simulink model "DTCFinal"  (R2017b)
settings: Solver=FixedStepDiscrete  StartTime=0.0  StopTime=60  FixedStep=Ts  MaxStep=Ts  RelTol=1e-3  EnableMultiTasking=on
InitFcn:
  | Vdc=560;Ts=2e-5;wb=2*pi*50;Rr=2.486;
  | Rs=4.125;Lls=0.01557;Llr=0.01557;Lm=0.2848;
  | Xls=4.8915;
  | Xlr=4.8915;
  | Xm=89.4726;
  | Xml=2.3807;
  | P=4;
  | J=0.139;
  | 
  | Kp=8;
  | Ki=35;
  | Tlim=15;
  | 
  | fc=3800;
  | F=0.001;
undefined symbols (not defined in the file): DiscIntNeverNeededParam
libraries: simulink x5, eeGeneralControl x2, powerlib x1
settings Model: Creator=Lenovo  LastModifiedBy=M.H
settings OptimizationCC: LifeSpan=inf
settings DebuggingCC: SFUnexpectedBacktrackingDiag=warning  SFNoUnconditionalDefaultTransitionDiag=warning  SFExecutionAtInitializationDiag=none
settings CodeAppCC: StateflowObjectComments=on
settings GRTTargetCC: TargetLangStandard=C89/C90 (ANSI)  GeneratePreprocessorConditionals=Disable all
settings ConfigComp: CovMetricSettings=dw  CovHtmlReporting=on  CovSaveCumulativeToWorkspaceVar=on  CovSaveSingleToWorkspaceVar=on  CovExternalEMLEnable=off

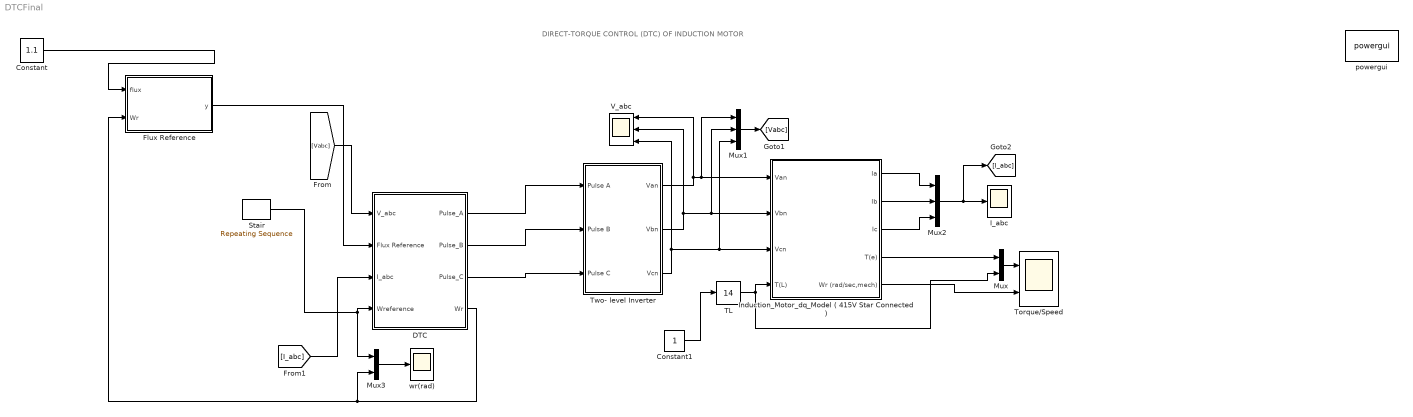
== system DTCFinal ==
  note: DIRECT-TORQUE CONTROL (DTC)
      | OF INDUCTION MOTOR
  Constant : Constant  Value=1.1
  Constant1 : Constant
  DTC : Subsystem
  Flux Reference : MATLAB Function  TreatAsAtomicUnit=on
  I_abc : Scope
  Induction_Motor_dq_Model ( 415V Star Connected ) : Subsystem
  Mux : Mux  Inputs=2
  Mux1 : Mux  Inputs=3
  Mux2 : Mux  Inputs=3
  Mux3 : Mux  Inputs=2
  "Stair " : simulink/Sources/Repeating Sequence  rep_seq_t=[0 0.1 0.11 4 4.1 8 8.1 12 12.1 16 18 19 20 22 22.5 23 25 26 29 30 35 40 50 55 60]  rep_seq_y=[0 0 10 10 20 20 30 30 40 40 60 80 100 110 120 130 140 150 160 170 200 300 400 400 400]
  TL : simulink/Math Operations/Slider Gain  gain=14  low=-14  high=14
  Torque/Speed : Scope  NumInputPorts=2
  "Two- level Inverter " : Subsystem
  V_abc : Scope  NumInputPorts=3
  powergui : powerlib/powergui  Priority=1  SimulationMode=Discrete  SampleTime=Ts  frequency=60  Iterations=50  frequencyindice=60  Pbase=100e6  ErrMax=1e-4  UnitsV=kV  UnitsW=MW  buscounter=0  FunctionMessages=off  echomessages=off  EnableUseOfTLC=off  CurrentSourceSwitches=off  DisableSnubberDevices=off  DisableRonSwitches=off  DisableVfSwitches=off  DisplayEquations=off  SolverType=Tustin/Backward Euler (TBE)  Interpol=off  ExternalGateDelay=off  methode=off  Ts=10  x0status=blocks  SPID=off  SwTol=0  HookPort=off  RestoreLinks=warning  ResistiveCurrentMeasurement=off  Frange=[0:2:500]  Ylog=off  Xlog=on  ShowGrid=off  save=off  variable=ZData  structure=ScopeData1  ZoomFFT=on  StartTime=0.0  cycles=4  DisplayStyle=2  fundamental=50  FreqAxis=off  MaxFrequency=1000  frequencyindicesteady=1  RmsSteady=1  display=off
  wr(rad) : Scope
  wires:
  Induction_Motor_dq_Model ( 415V Star Connected )/1(Ia) -> Mux2/1
  Induction_Motor_dq_Model ( 415V Star Connected )/2(Ib) -> Mux2/2
  Induction_Motor_dq_Model ( 415V Star Connected )/3(Ic) -> Mux2/3
  Induction_Motor_dq_Model ( 415V Star Connected )/5(Wr (rad/sec,mech)) -> Torque/Speed/2
  "Two- level Inverter "/1(Van) -> V_abc/1, Mux1/1, Induction_Motor_dq_Model ( 415V Star Connected )/1(Van)
  "Two- level Inverter "/3(Vcn) -> V_abc/3, Mux1/3, Induction_Motor_dq_Model ( 415V Star Connected )/3(Vcn)
  "Two- level Inverter "/2(Vbn) -> V_abc/2, Mux1/2, Induction_Motor_dq_Model ( 415V Star Connected )/2(Vbn)
  TL/1 -> Mux/2, Induction_Motor_dq_Model ( 415V Star Connected )/4(T(L))
  Constant1/1 -> TL/1
  Induction_Motor_dq_Model ( 415V Star Connected )/4(T(e)) -> Mux/1
  Mux/1 -> Torque/Speed/1
  Mux2/1 -> [I_abc], I_abc/1
  DTC/1(Pulse_A) -> "Two- level Inverter "/1(Pulse A)
  DTC/3(Pulse_C) -> "Two- level Inverter "/3(Pulse C)
  DTC/2(Pulse_B) -> "Two- level Inverter "/2(Pulse B)
  Mux1/1 -> [Vabc]
  Mux3/1 -> wr(rad)/1
  [Vabc] -> DTC/1(V_abc)
  [I_abc] -> DTC/3(I_abc)
  Flux Reference/1(y) -> DTC/2(Flux Reference)
  DTC/4(Wr) -> Flux Reference/2(Wr), Mux3/2
  Constant/1 -> Flux Reference/1(flux)
  "Stair "/1 -> Mux3/1, DTC/4(Wreference)

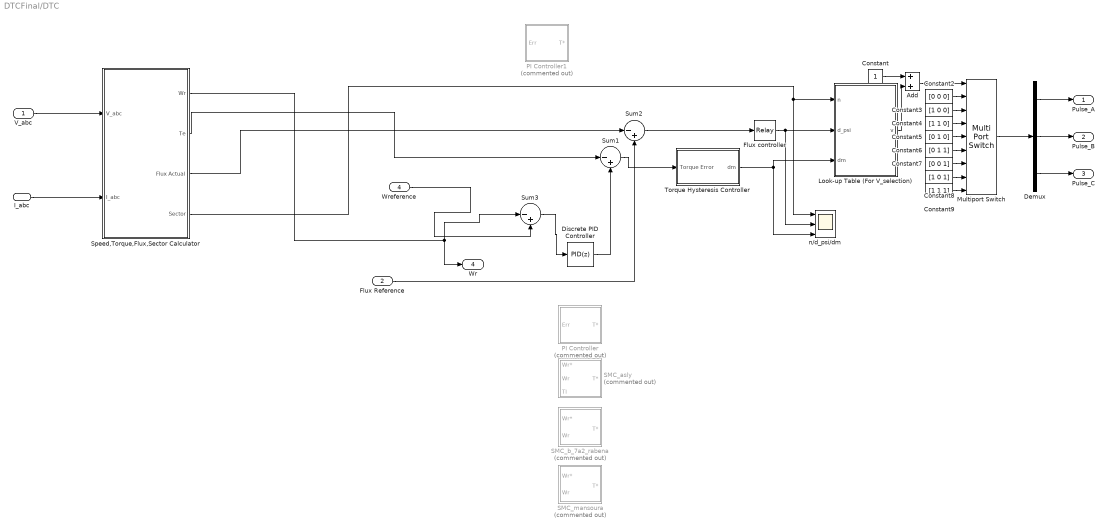
== system DTCFinal/DTC ==
  V_abc : Inport
  Flux Reference : Inport  Port=2
  I_abc : Inport  Port=3
  Wreference : Inport  Port=4
  Add : Sum
  Constant : Constant
  Constant2 : Constant  Value=[0 0 0]
  Constant3 : Constant  Value=[1 0 0]
  Constant4 : Constant  Value=[1 1 0]
  Constant5 : Constant  Value=[0 1 0]
  Constant6 : Constant  Value=[0 1 1]
  Constant7 : Constant  Value=[0 0 1]
  Constant8 : Constant  Value=[1 0 1]
  Constant9 : Constant  Value=[1 1 1]
  Demux : Demux  Outputs=3
  Discrete PID Controller : simulink/Continuous/PID Controller  Controller=PID  TimeDomain=Discrete-time  SampleTime=-1  IntegratorMethod=Forward Euler  FilterMethod=Forward Euler  Form=Parallel  UseFilter=on  ControllerParametersSource=internal  P=10  I=2  D=0  N=100  InitialConditionSource=internal  InitialConditionForIntegrator=0  InitialConditionForFilter=0  ExternalReset=none  LimitOutput=off  UpperSaturationLimit=inf  LowerSaturationLimit=-inf  LinearizeAsGain=off  AntiWindupMode=none  Kb=1  TrackingMode=off  Kt=1  PParamMin=[]  PParamMax=[]  IParamMin=[]  IParamMax=[]  DParamMin=[]  DParamMax=[]  NParamMin=[]  NParamMax=[]  KbParamMin=[]  KbParamMax=[]  KtParamMin=[]  KtParamMax=[]  POutMin=[]  POutMax=[]  IOutMin=[]  IOutMax=[]  DOutMin=[]  DOutMax=[]  NOutMin=[]  NOutMax=[]  KbOutMin=[]  KbOutMax=[]  KtOutMin=[]  KtOutMax=[]  IntegratorOutMin=[]  IntegratorOutMax=[]  FilterOutMin=[]  FilterOutMax=[]  SumOutMin=[]  SumOutMax=[]  SumI1OutMin=[]  SumI1OutMax=[]  SumI2OutMin=[]  SumI2OutMax=[]  SumI3OutMin=[]  SumI3OutMax=[]  SumDOutMin=[]  SumDOutMax=[]  SaturationOutMin=[]  SaturationOutMax=[]  IntegratorContinuousStateAttributes=''  IntegratorStateMustResolveToSignalObject=off  IntegratorRTWStateStorageClass=Auto  FilterContinuousStateAttributes=''  FilterStateMustResolveToSignalObject=off  FilterRTWStateStorageClass=Auto  DifferentiatorICPrevScaledInput=0  DifferentiatorOutMin=[]  DifferentiatorOutMax=[]  InitialConditionSetting=State (most efficient)  FilterDiffOutCoefMin=[]  FilterDiffOutCoefMax=[]  SumDenOutMin=[]  SumDenOutMax=[]  SumNumOutMin=[]  SumNumOutMax=[]  ReciprocalOutMin=[]  ReciprocalOutMax=[]  DivideOutMin=[]  DivideOutMax=[]  TunerSelectOption=Transfer Function Based (PID Tuner App)
  Flux controller : Relay  OnSwitchValue=0.02  OffSwitchValue=-0.02
  Look-up Table (For V_selection) : MATLAB Function  TreatAsAtomicUnit=on
  Multiport Switch : MultiPortSwitch  Inputs=8
  PI Controller : Subsystem  Commented=on
  PI Controller1 : Subsystem  Commented=on
  "SMC_asly " : Subsystem  Commented=on
  "SMC_b_7a2_rabena " : Subsystem  Commented=on
  "SMC_mansoura " : Subsystem  Commented=on
  Speed,Torque,Flux,Sector Calculator : Subsystem
  Sum1 : Sum  Inputs=|-+
  Sum2 : Sum  Inputs=|-+
  Sum3 : Sum  Inputs=|-+
  Torque Hysteresis Controller : Subsystem
  n/d_psi/dm : Scope  NumInputPorts=3
  Pulse_A : Outport
  Pulse_B : Outport  Port=2
  Pulse_C : Outport  Port=3
  Wr : Outport  Port=4
  wires:
  Flux controller/1 -> Look-up Table (For V_selection)/2(d_psi), n/d_psi/dm/2
  Sum2/1 -> Flux controller/1
  Speed,Torque,Flux,Sector Calculator/4(Sector) -> n/d_psi/dm/1, Look-up Table (For V_selection)/1(n)
  Torque Hysteresis Controller/1(dm) -> Look-up Table (For V_selection)/3(dm), n/d_psi/dm/3
  Flux Reference/1 -> Sum2/2
  Add/1 -> Multiport Switch/1
  Sum1/1 -> Torque Hysteresis Controller/1(Torque Error)
  Constant9/1 -> Multiport Switch/9
  Constant6/1 -> Multiport Switch/6
  Constant2/1 -> Multiport Switch/2
  Constant3/1 -> Multiport Switch/3
  Constant5/1 -> Multiport Switch/5
  Demux/3 -> Pulse_C/1
  Constant8/1 -> Multiport Switch/8
  Look-up Table (For V_selection)/1(v) -> Add/2
  Constant/1 -> Add/1
  Demux/1 -> Pulse_A/1
  Demux/2 -> Pulse_B/1
  Constant7/1 -> Multiport Switch/7
  Constant4/1 -> Multiport Switch/4
  Multiport Switch/1 -> Demux/1
  V_abc/1 -> Speed,Torque,Flux,Sector Calculator/1(V_abc)
  I_abc/1 -> Speed,Torque,Flux,Sector Calculator/2(I_abc)
  Speed,Torque,Flux,Sector Calculator/2(Te) -> Sum1/1
  Speed,Torque,Flux,Sector Calculator/3(Flux Actual) -> Sum2/1
  Speed,Torque,Flux,Sector Calculator/1(Wr) -> Sum3/1, Wr/1
  Wreference/1 -> Sum3/2
  Sum3/1 -> Discrete PID Controller/1
  Discrete PID Controller/1 -> Sum1/2

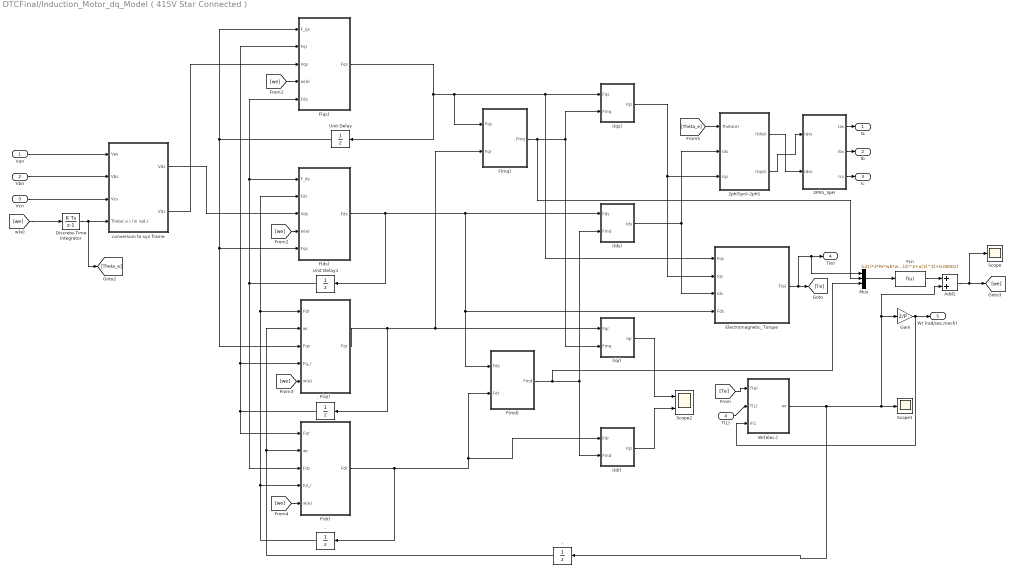
== system DTCFinal/Induction_Motor_dq_Model ( 415V Star Connected ) ==
  Van : Inport
  Vbn : Inport  Port=2
  Vcn : Inport  Port=3
  T(L) : Inport  Port=4
  . : UnitDelay  SampleTime=Ts
  ". " : UnitDelay  SampleTime=Ts
  ".  " : UnitDelay  SampleTime=Ts
  2PhS_3pH : Subsystem
  2ph(Syn)-2phS : Subsystem
  Add1 : Sum
  Discrete-Time Integrator : DiscreteIntegrator  InitialConditionSetting=State (most efficient)  SampleTime=Ts  ICPrevOutput=DiscIntNeverNeededParam  ICPrevScaledInput=DiscIntNeverNeededParam
  Electromagnetic_Torque : Subsystem
  F(dr) : Subsystem
  F(ds) : Subsystem
  F(md) : Subsystem
  F(mq) : Subsystem
  F(qr) : Subsystem
  F(qs) : Subsystem
  Fcn : Fcn  Expr=(u(1)*2*Rr*wb*wb)/(3*P*(u(2)^2+u(3)^2)+0.00001)
  Gain : Gain  Gain=2/P
  I(dr) : Subsystem
  I(ds) : Subsystem
  I(qr) : Subsystem
  I(qs) : Subsystem
  Mux : Mux  Inputs=3
  Scope : Scope
  Scope1 : Scope
  Scope2 : Scope  NumInputPorts=2
  Unit Delay : UnitDelay  SampleTime=Ts
  Unit Delay1 : UnitDelay  SampleTime=Ts
  Wr(elec.) : Subsystem
  "conversion to syn frame " : Subsystem
  Ia : Outport
  Ib : Outport  Port=2
  Ic : Outport  Port=3
  T(e) : Outport  Port=4
  Wr (rad/sec,mech) : Outport  Port=5
  wires:
  F(mq)/1(Fmq) -> Mux/2, I(qs)/2(Fmq), I(qr)/2(Fmq)
  I(ds)/1(Ids) -> Electromagnetic_Torque/3(Ids), 2ph(Syn)-2phS/2(Ids)
  I(qs)/1(Iqs) -> Electromagnetic_Torque/2(Iqs), 2ph(Syn)-2phS/3(Iqs)
  Wr(elec.)/1(wr) -> Scope1/1, Gain/1, Add1/2, ".  "/1
  Van/1 -> "conversion to syn frame "/1(Vas)
  I(dr)/1(Iqs) -> Scope2/2
  "conversion to syn frame "/1(Vds) -> F(ds)/3(Vds)
  Vcn/1 -> "conversion to syn frame "/3(Vcs)
  Vbn/1 -> "conversion to syn frame "/2(Vbs)
  "conversion to syn frame "/2(Vqs) -> F(qs)/3(Vqs)
  F(dr)/1(Fdr) -> ". "/1, F(md)/2(Fdr), I(dr)/1("Fdr ")
  F(ds)/1(Fds) -> Unit Delay1/1, I(ds)/1("Fds "), Electromagnetic_Torque/4(Fds), F(md)/1(Fds)
  F(qr)/1(Fqr) -> ./1, I(qr)/1("Fqr "), F(mq)/2(Fqr)
  I(qr)/1(Iqr) -> Scope2/1
  2ph(Syn)-2phS/1(I(dss)) -> 2PhS_3pH/2(Idss)
  2ph(Syn)-2phS/2(I(qss)) -> 2PhS_3pH/1(Iqss)
  F(qs)/1(Fqs) -> Unit Delay/1, Electromagnetic_Torque/1(Fqs), I(qs)/1("Fqs "), F(mq)/1(Fqs)
  [we] -> Discrete-Time Integrator/1
  [Theta_e] -> 2ph(Syn)-2phS/1(Theta(e))
  [we] -> F(dr)/5(w(e))
  Electromagnetic_Torque/1(T(e)) -> Mux/1, T(e)/1, [Te]
  2PhS_3pH/3(Ics) -> Ic/1
  T(L)/1 -> Wr(elec.)/2(T(L))
  2PhS_3pH/1(Ias) -> Ia/1
  2PhS_3pH/2(Ibs) -> Ib/1
  [we] -> F(qs)/4("w(e) ")
  [Te] -> Wr(elec.)/1(T(e))
  [we] -> F(qr)/5(w(e))
  [we] -> F(ds)/4("w(e) ")
  Discrete-Time Integrator/1 -> "conversion to syn frame "/4("Theta( e ) (in rad.) "), [Theta_e]
  Unit Delay/1 -> F(qs)/1(F_qs), F(ds)/5(Fqs), F(qr)/3(Fqs)
  Unit Delay1/1 -> F(ds)/1(F_ds), F(qs)/5(Fds), F(dr)/3(Fds)
  ./1 -> F(dr)/1(Fqr), F(qr)/4(Fq_r), F(qs)/2(Fqr)
  ". "/1 -> F(ds)/2(Fdr), F(qr)/1(Fdr), F(dr)/4(Fd_r)
  ".  "/1 -> F(qr)/2(wr), F(dr)/2(wr)
  F(md)/1(Fmd) -> Mux/3, I(ds)/2(Fmd), I(dr)/2(Fmd)
  Fcn/1 -> Add1/1
  Add1/1 -> Scope/1, [we]
  Mux/1 -> Fcn/1
  Gain/1 -> Wr(elec.)/3(In1), Wr (rad/sec,mech)/1

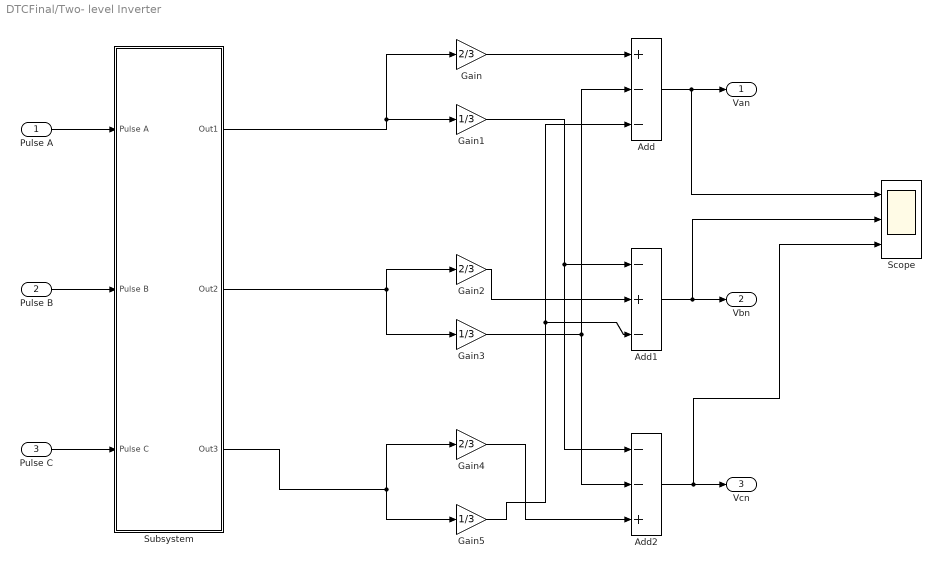
== system DTCFinal/Two- level Inverter  ==
  Pulse A : Inport
  Pulse B : Inport  Port=2
  Pulse C : Inport  Port=3
  Add : Sum  Inputs=+--
  Add1 : Sum  Inputs=-+-
  Add2 : Sum  Inputs=--+
  Gain : Gain  Gain=2/3
  Gain1 : Gain  Gain=1/3
  Gain2 : Gain  Gain=2/3
  Gain3 : Gain  Gain=1/3
  Gain4 : Gain  Gain=2/3
  Gain5 : Gain  Gain=1/3
  Scope : Scope  NumInputPorts=3
  Subsystem : Subsystem
  Van : Outport
  Vbn : Outport  Port=2
  Vcn : Outport  Port=3
  wires:
  Pulse C/1 -> Subsystem/3(Pulse C)
  Pulse B/1 -> Subsystem/2(Pulse B)
  Pulse A/1 -> Subsystem/1(Pulse A)
  Subsystem/2(Out2) -> Gain3/1, Gain2/1
  Subsystem/3(Out3) -> Gain4/1, Gain5/1
  Subsystem/1(Out1) -> Gain1/1, Gain/1
  Gain4/1 -> Add2/3
  Add/1 -> Scope/1, Van/1
  Add2/1 -> Vcn/1, Scope/3
  Gain3/1 -> Add/2, Add2/2
  Add1/1 -> Vbn/1, Scope/2
  Gain5/1 -> Add1/3, Add/3
  Gain/1 -> Add/1
  Gain2/1 -> Add1/2
  Gain1/1 -> Add1/1, Add2/1

== system DTCFinal/DTC/PI Controller ==
  Err : Inport
  "Integrator " : DiscreteIntegrator  InitialConditionSetting=State (most efficient)  SampleTime=Ts  LimitOutput=on  UpperSaturationLimit=Tlim  LowerSaturationLimit=-Tlim  ICPrevOutput=DiscIntNeverNeededParam  ICPrevScaledInput=DiscIntNeverNeededParam
  Ki : Gain  Gain=Ki
  Kp : Gain  Gain=Kp
  Saturation : Saturate  UpperLimit=Tlim  LowerLimit=-Tlim
  Sum1 : Sum  Inputs=|++
  T* : Outport
  wires:
  Err/1 -> Ki/1, Kp/1
  Ki/1 -> "Integrator "/1
  Kp/1 -> Sum1/1
  "Integrator "/1 -> Sum1/2
  Sum1/1 -> Saturation/1
  Saturation/1 -> T*/1

== system DTCFinal/DTC/PI Controller1 ==
  Err : Inport
  "Integrator " : DiscreteIntegrator  InitialConditionSetting=State (most efficient)  SampleTime=Ts  LimitOutput=on  UpperSaturationLimit=Tlim  LowerSaturationLimit=-Tlim  ICPrevOutput=DiscIntNeverNeededParam  ICPrevScaledInput=DiscIntNeverNeededParam
  Ki : Gain  Gain=Ki
  Kp : Gain  Gain=Kp
  Saturation : Saturate  UpperLimit=Tlim  LowerLimit=-Tlim
  Sum1 : Sum  Inputs=|++
  T* : Outport
  wires:
  Err/1 -> Ki/1, Kp/1
  Ki/1 -> "Integrator "/1
  Kp/1 -> Sum1/1
  "Integrator "/1 -> Sum1/2
  Sum1/1 -> Saturation/1
  Saturation/1 -> T*/1

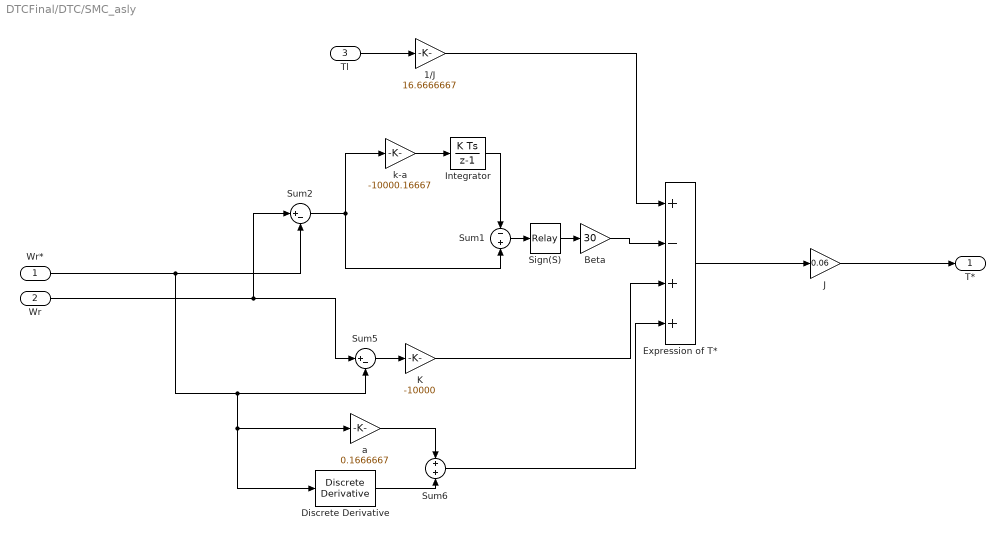
== system DTCFinal/DTC/SMC_asly  ==
  "Wr* " : Inport
  Wr : Inport  Port=2
  "Tl " : Inport  Port=3
  1/J : Gain  Gain=16.6666667
  Beta : Gain  Gain=30
  Discrete Derivative : simulink/Discrete/Discrete Derivative  gainval=1  ICPrevScaledInput=0.0  OutMin=[]  OutMax=[]  OutDataType=fixdt(1, 16)  OutScaling=2^-10  DoSatur=off
  "Expression of T* " : Sum  Inputs=+-++
  "Integrator " : DiscreteIntegrator  gainval=1  InitialConditionSetting=State (most efficient)  SampleTime=Ts  LimitOutput=on  UpperSaturationLimit=Tlim  LowerSaturationLimit=-Tlim  ICPrevOutput=DiscIntNeverNeededParam  ICPrevScaledInput=DiscIntNeverNeededParam
  J : Gain  Gain=0.06
  "K " : Gain  Gain=-10000
  Sign(S) : Relay  OnSwitchValue=0.02  OffSwitchValue=-0.02
  Sum1 : Sum  Inputs=-|+
  Sum2 : Sum  Inputs=|+-
  Sum5 : Sum  Inputs=|+-
  Sum6 : Sum  Inputs=+|+
  a : Gain  Gain=0.1666667
  k-a : Gain  Gain=-10000.16667
  T* : Outport
  wires:
  Sum2/1 -> k-a/1, Sum1/2
  Sum1/1 -> Sign(S)/1
  "Expression of T* "/1 -> J/1
  "Integrator "/1 -> Sum1/1
  Wr/1 -> Sum5/1, Sum2/1
  J/1 -> T*/1
  k-a/1 -> "Integrator "/1
  Sign(S)/1 -> Beta/1
  Sum5/1 -> "K "/1
  "K "/1 -> "Expression of T* "/3
  a/1 -> Sum6/1
  Discrete Derivative/1 -> Sum6/2
  Sum6/1 -> "Expression of T* "/4
  "Tl "/1 -> 1/J/1
  "Wr* "/1 -> Sum2/2, a/1, Discrete Derivative/1, Sum5/2
  1/J/1 -> "Expression of T* "/1
  Beta/1 -> "Expression of T* "/2

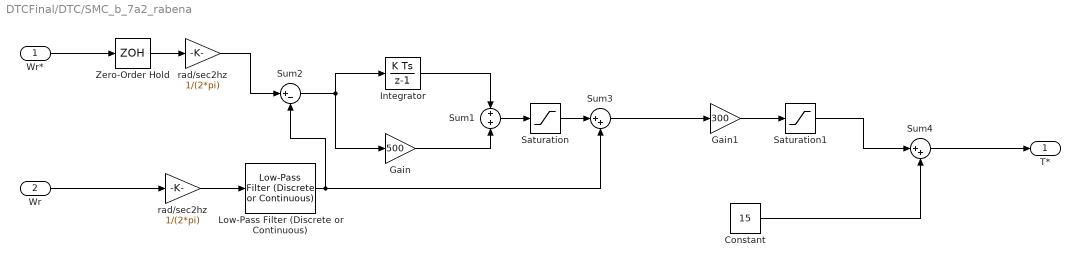
== system DTCFinal/DTC/SMC_b_7a2_rabena  ==
  "Wr* " : Inport
  Wr : Inport  Port=2
  Constant : Constant  Value=15
  Gain : Gain  Gain=500
  Gain1 : Gain  Gain=300
  "Integrator " : DiscreteIntegrator  gainval=1  InitialConditionSetting=State (most efficient)  SampleTime=Ts  LimitOutput=on  UpperSaturationLimit=Tlim  LowerSaturationLimit=-Tlim  ICPrevOutput=DiscIntNeverNeededParam  ICPrevScaledInput=DiscIntNeverNeededParam
  Low-Pass Filter (Discrete or Continuous) : eeGeneralControl/Low-Pass Filter (Discrete or Continuous)  K=1  T=0.0025  B=inf  A=-inf  Ts=-1
      settings: SourceProductName=Simscape Electrical
  Saturation : Saturate  UpperLimit=Tlim  LowerLimit=-Tlim
  Saturation1 : Saturate  UpperLimit=Tlim  LowerLimit=-Tlim
  Sum1 : Sum  Inputs=+|+
  Sum2 : Sum  Inputs=|+-
  Sum3 : Sum  Inputs=|++
  Sum4 : Sum  Inputs=|++
  Zero-Order Hold : ZeroOrderHold  SampleTime=-1
  "rad/sec2hz " : Gain  Gain=1/(2*pi)
  "rad/sec2hz " : Gain  Gain=1/(2*pi)
  T* : Outport
  wires:
  "Wr* "/1 -> Zero-Order Hold/1
  Zero-Order Hold/1 -> "rad/sec2hz "/1
  Wr/1 -> "rad/sec2hz "/1
  "rad/sec2hz "/1 -> Sum2/1
  Gain/1 -> Sum1/2
  Sum1/1 -> Saturation/1
  Saturation/1 -> Sum3/1
  Sum3/1 -> Gain1/1
  Gain1/1 -> Saturation1/1
  Sum2/1 -> "Integrator "/1, Gain/1
  "Integrator "/1 -> Sum1/1
  "rad/sec2hz "/1 -> Low-Pass Filter (Discrete or Continuous)/1
  Low-Pass Filter (Discrete or Continuous)/1 -> Sum3/2, Sum2/2
  Saturation1/1 -> Sum4/1
  Sum4/1 -> T*/1
  Constant/1 -> Sum4/2

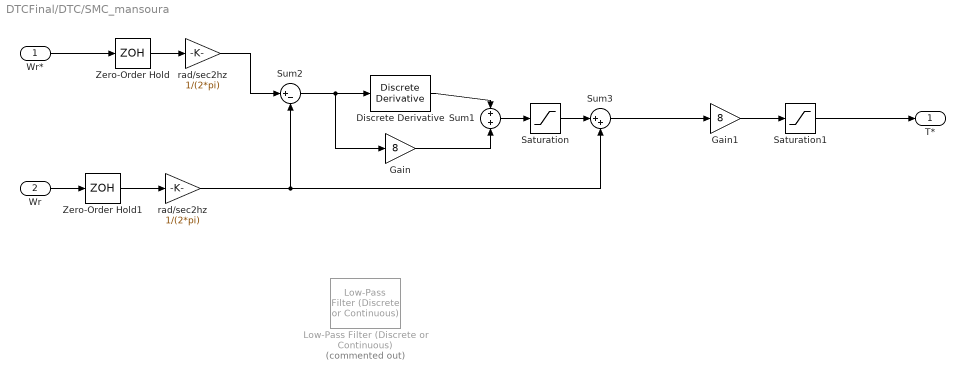
== system DTCFinal/DTC/SMC_mansoura  ==
  "Wr* " : Inport
  Wr : Inport  Port=2
  Discrete Derivative : simulink/Discrete/Discrete Derivative  gainval=1.0  ICPrevScaledInput=0.0  OutMin=[]  OutMax=[]  OutDataType=fixdt(1, 16)  OutScaling=2^-10  DoSatur=off
  Gain : Gain  Gain=8
  Gain1 : Gain  Gain=8
  Low-Pass Filter (Discrete or Continuous) : eeGeneralControl/Low-Pass Filter (Discrete or Continuous)  Commented=on  K=2  T=1  B=inf  A=-inf  Ts=-1
      settings: SourceProductName=Simscape Electrical
  Saturation : Saturate  UpperLimit=Tlim  LowerLimit=-Tlim
  Saturation1 : Saturate  UpperLimit=Tlim  LowerLimit=-Tlim
  Sum1 : Sum  Inputs=+|+
  Sum2 : Sum  Inputs=|+-
  Sum3 : Sum  Inputs=|++
  Zero-Order Hold : ZeroOrderHold  SampleTime=-1
  Zero-Order Hold1 : ZeroOrderHold  SampleTime=-1
  "rad/sec2hz " : Gain  Gain=1/(2*pi)
  "rad/sec2hz " : Gain  Gain=1/(2*pi)
  T* : Outport
  wires:
  "Wr* "/1 -> Zero-Order Hold/1
  Zero-Order Hold/1 -> "rad/sec2hz "/1
  Wr/1 -> Zero-Order Hold1/1
  Zero-Order Hold1/1 -> "rad/sec2hz "/1
  "rad/sec2hz "/1 -> Sum2/1
  "rad/sec2hz "/1 -> Sum3/2, Sum2/2
  Sum2/1 -> Discrete Derivative/1, Gain/1
  Gain/1 -> Sum1/2
  Sum1/1 -> Saturation/1
  Saturation/1 -> Sum3/1
  Sum3/1 -> Gain1/1
  Gain1/1 -> Saturation1/1
  Saturation1/1 -> T*/1
  Discrete Derivative/1 -> Sum1/1

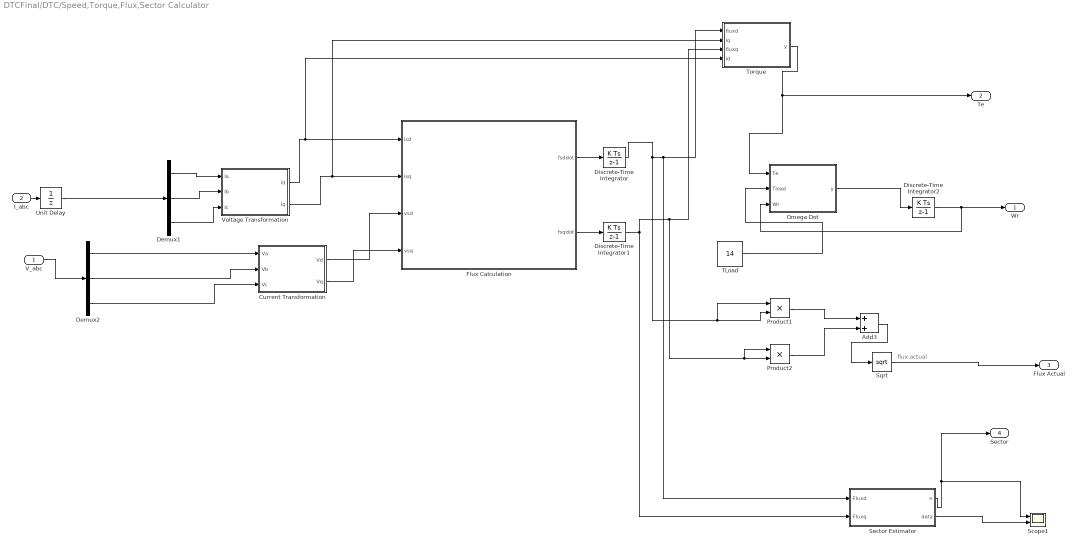
== system DTCFinal/DTC/Speed,Torque,Flux,Sector Calculator ==
  note: flux actual
  V_abc : Inport
  I_abc : Inport  Port=2
  Add3 : Sum
  Current Transformation : MATLAB Function  TreatAsAtomicUnit=on
  Demux1 : Demux  Outputs=3
  Demux2 : Demux  Outputs=3
  Discrete-Time Integrator : DiscreteIntegrator  InitialConditionSetting=State (most efficient)  SampleTime=-1  ICPrevOutput=DiscIntNeverNeededParam  ICPrevScaledInput=DiscIntNeverNeededParam
  Discrete-Time Integrator1 : DiscreteIntegrator  InitialConditionSetting=State (most efficient)  SampleTime=-1  ICPrevOutput=DiscIntNeverNeededParam  ICPrevScaledInput=DiscIntNeverNeededParam
  Discrete-Time Integrator2 : DiscreteIntegrator  InitialConditionSetting=State (most efficient)  SampleTime=-1  ICPrevOutput=DiscIntNeverNeededParam  ICPrevScaledInput=DiscIntNeverNeededParam
  Flux Calculation : MATLAB Function  TreatAsAtomicUnit=on
  Omega Dot : MATLAB Function  TreatAsAtomicUnit=on
  Product1 : Product
  Product2 : Product
  Scope1 : Scope  NumInputPorts=2
  Sector Estimator : MATLAB Function  TreatAsAtomicUnit=on
  Sqrt : Sqrt  SaturateOnIntegerOverflow=on
  TLoad : Constant  Value=14  VectorParams1D=off  SampleTime=-1
  Torque : MATLAB Function  TreatAsAtomicUnit=on
  Unit Delay : UnitDelay  SampleTime=-1
  Voltage Transformation : MATLAB Function  TreatAsAtomicUnit=on
  Wr : Outport
  Te : Outport  Port=2
  Flux Actual : Outport  Port=3
  Sector : Outport  Port=4
  wires:
  Flux Calculation/2(fsqdot) -> Discrete-Time Integrator1/1
  TLoad/1 -> Omega Dot/2(Tload)
  Flux Calculation/1(fsddot) -> Discrete-Time Integrator/1
  Torque/1(y) -> Te/1, Omega Dot/1(Te)
  Demux1/2 -> Voltage Transformation/2(Ib)
  Demux1/1 -> Voltage Transformation/1(Ia)
  Omega Dot/1(y) -> Discrete-Time Integrator2/1
  I_abc/1 -> Unit Delay/1
  Demux2/2 -> Current Transformation/2(Vb)
  V_abc/1 -> Demux2/1
  Demux2/3 -> Current Transformation/3(Vc)
  Demux2/1 -> Current Transformation/1(Va)
  Unit Delay/1 -> Demux1/1
  Current Transformation/2(Vq) -> Flux Calculation/4(vsq)
  Voltage Transformation/2(Iq) -> Torque/2(iq), Flux Calculation/2(isq)
  Current Transformation/1(Vd) -> Flux Calculation/3(vsd)
  Demux1/3 -> Voltage Transformation/3(Ic)
  Voltage Transformation/1(Id) -> Torque/4(id), Flux Calculation/1(isd)
  Discrete-Time Integrator2/1 -> Omega Dot/3(Wr), Wr/1
  Add3/1 -> Sqrt/1
  Sqrt/1 -> Flux Actual/1
  Discrete-Time Integrator1/1 -> Sector Estimator/2(Fluxq), Product2/1, Product2/2, Torque/3(fluxq)
  Product2/1 -> Add3/2
  Product1/1 -> Add3/1
  Sector Estimator/2(deta) -> Scope1/2
  Sector Estimator/1(n) -> Sector/1, Scope1/1
  Discrete-Time Integrator/1 -> Product1/2, Product1/1, Sector Estimator/1(Fluxd), Torque/1(fluxd)

== system DTCFinal/DTC/Torque Hysteresis Controller ==
  Torque Error : Inport
  Add : Sum
  Flux controller1 : Relay  OnSwitchValue=0.2  OffSwitchValue=0
  Flux controller2 : Relay  OnSwitchValue=0  OffSwitchValue=-0.2  OnOutputValue=0  OffOutputValue=-1
  dm : Outport
  wires:
  Add/1 -> dm/1
  Flux controller2/1 -> Add/2
  Flux controller1/1 -> Add/1
  Torque Error/1 -> Flux controller2/1, Flux controller1/1

== system DTCFinal/Induction_Motor_dq_Model ( 415V Star Connected )/2PhS_3pH ==
  Iqss : Inport
  Idss : Inport  Port=2
  Add : Sum
  Add1 : Sum
  Gain : Gain  Gain=-0.5
  Gain1 : Gain  Gain=-1.732/2
  Gain2 : Gain  Gain=-0.5
  Gain3 : Gain  Gain=1.732/2
  Ias : Outport
  Ibs : Outport  Port=2
  Ics : Outport  Port=3
  wires:
  Gain3/1 -> Add1/2
  Add/1 -> Ibs/1
  Gain2/1 -> Add1/1
  Add1/1 -> Ics/1
  Gain1/1 -> Add/2
  Gain/1 -> Add/1
  Idss/1 -> Gain3/1, Gain1/1
  Iqss/1 -> Ias/1, Gain2/1, Gain/1

== system DTCFinal/Induction_Motor_dq_Model ( 415V Star Connected )/2ph(Syn)-2phS ==
  Theta(e) : Inport
  Ids : Inport  Port=2
  Iqs : Inport  Port=3
  Idss : Sum  Inputs=+-
  Iqss : Sum
  Product{,1..3} (4 alike) : Product
  T : Trigonometry  Operator=cos
  T1 : Trigonometry
  T2 : Trigonometry
  T3 : Trigonometry  Operator=cos
  I(dss) : Outport
  I(qss) : Outport  Port=2
  wires:
  T/1 -> Product/1
  Product/1 -> Idss/1
  Product1/1 -> Idss/2
  Idss/1 -> I(dss)/1
  Iqss/1 -> I(qss)/1
  T1/1 -> Product1/1
  T2/1 -> Product2/1
  Iqs/1 -> Product3/2, Product1/2
  Product3/1 -> Iqss/2
  Theta(e)/1 -> T3/1, T2/1, T1/1, T/1
  Ids/1 -> Product/2, Product2/2
  Product2/1 -> Iqss/1
  T3/1 -> Product3/1

== system DTCFinal/Induction_Motor_dq_Model ( 415V Star Connected )/Electromagnetic_Torque ==
  Fqs : Inport
  Iqs : Inport  Port=2
  Ids : Inport  Port=3
  Fds : Inport  Port=4
  Add : Sum  Inputs=+-
  Gain : Gain  Gain=(3*P)/(4*wb)
  Product : Product
  Product1 : Product
  T(e) : Outport
  wires:
  Gain/1 -> T(e)/1
  Fds/1 -> Product/1
  Fqs/1 -> Product1/1
  Ids/1 -> Product1/2
  Iqs/1 -> Product/2
  Product/1 -> Add/1
  Add/1 -> Gain/1
  Product1/1 -> Add/2

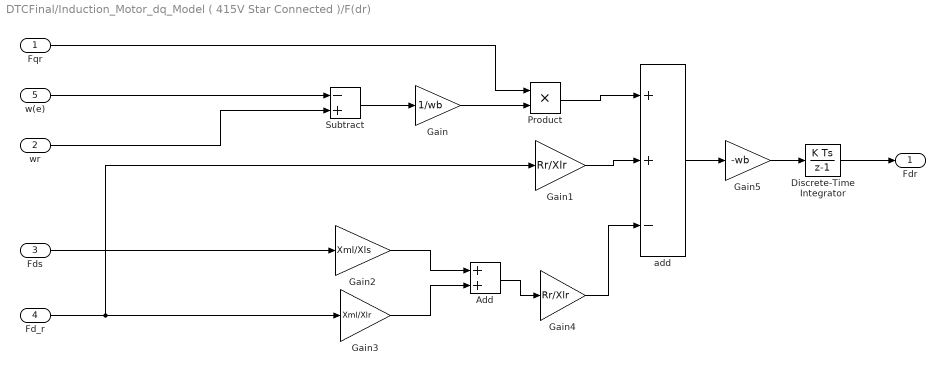
== system DTCFinal/Induction_Motor_dq_Model ( 415V Star Connected )/F(dr) ==
  Fqr : Inport
  wr : Inport  Port=2
  Fds : Inport  Port=3
  Fd_r : Inport  Port=4
  w(e) : Inport  Port=5
  Add : Sum
  Discrete-Time Integrator : DiscreteIntegrator  InitialConditionSetting=State (most efficient)  SampleTime=Ts  ICPrevOutput=DiscIntNeverNeededParam  ICPrevScaledInput=DiscIntNeverNeededParam
  Gain : Gain  Gain=1/wb
  Gain1 : Gain  Gain=Rr/Xlr
  Gain2 : Gain  Gain=Xml/Xls
  Gain3 : Gain  Gain=Xml/Xlr
  Gain4 : Gain  Gain=Rr/Xlr
  Gain5 : Gain  Gain=-wb
  Product : Product
  Subtract : Sum  Inputs=-+
  add : Sum  Inputs=++-
  Fdr : Outport
  wires:
  Discrete-Time Integrator/1 -> Fdr/1
  Gain5/1 -> Discrete-Time Integrator/1
  add/1 -> Gain5/1
  w(e)/1 -> Subtract/1
  Subtract/1 -> Gain/1
  Add/1 -> Gain4/1
  Fds/1 -> Gain2/1
  Gain2/1 -> Add/1
  Gain3/1 -> Add/2
  Gain/1 -> Product/2
  wr/1 -> Subtract/2
  Gain1/1 -> add/2
  Gain4/1 -> add/3
  Fd_r/1 -> Gain3/1, Gain1/1
  Fqr/1 -> Product/1
  Product/1 -> add/1

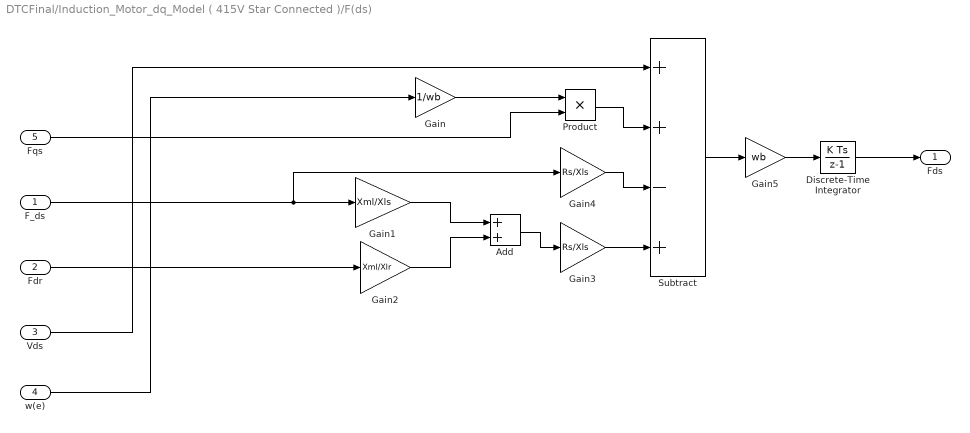
== system DTCFinal/Induction_Motor_dq_Model ( 415V Star Connected )/F(ds) ==
  F_ds : Inport
  Fdr : Inport  Port=2
  Vds : Inport  Port=3
  "w(e) " : Inport  Port=4
  Fqs : Inport  Port=5
  Add : Sum
  Discrete-Time Integrator : DiscreteIntegrator  InitialConditionSetting=State (most efficient)  SampleTime=Ts  ICPrevOutput=DiscIntNeverNeededParam  ICPrevScaledInput=DiscIntNeverNeededParam
  Gain : Gain  Gain=1/wb
  Gain1 : Gain  Gain=Xml/Xls
  Gain2 : Gain  Gain=Xml/Xlr
  Gain3 : Gain  Gain=Rs/Xls
  Gain4 : Gain  Gain=Rs/Xls
  Gain5 : Gain  Gain=wb
  Product : Product
  Subtract : Sum  Inputs=++-+
  Fds : Outport
  wires:
  Gain/1 -> Product/1
  Vds/1 -> Subtract/1
  Gain2/1 -> Add/2
  Discrete-Time Integrator/1 -> Fds/1
  Subtract/1 -> Gain5/1
  Gain5/1 -> Discrete-Time Integrator/1
  Product/1 -> Subtract/2
  Fqs/1 -> Product/2
  Add/1 -> Gain3/1
  Gain3/1 -> Subtract/4
  Gain4/1 -> Subtract/3
  F_ds/1 -> Gain1/1, Gain4/1
  Gain1/1 -> Add/1
  Fdr/1 -> Gain2/1
  "w(e) "/1 -> Gain/1

== system DTCFinal/Induction_Motor_dq_Model ( 415V Star Connected )/F(md) ==
  Fds : Inport
  Fdr : Inport  Port=2
  Add : Sum
  Gain1 : Gain  Gain=Xml/Xls
  Gain2 : Gain  Gain=Xml/Xlr
  Fmd : Outport
  wires:
  Add/1 -> Fmd/1
  Fds/1 -> Gain1/1
  Fdr/1 -> Gain2/1
  Gain2/1 -> Add/2
  Gain1/1 -> Add/1

== system DTCFinal/Induction_Motor_dq_Model ( 415V Star Connected )/F(mq) ==
  Fqs : Inport
  Fqr : Inport  Port=2
  Add : Sum
  Gain1 : Gain  Gain=Xml/Xls
  Gain2 : Gain  Gain=Xml/Xlr
  Fmq : Outport
  wires:
  Gain1/1 -> Add/1
  Gain2/1 -> Add/2
  Fqr/1 -> Gain2/1
  Fqs/1 -> Gain1/1
  Add/1 -> Fmq/1

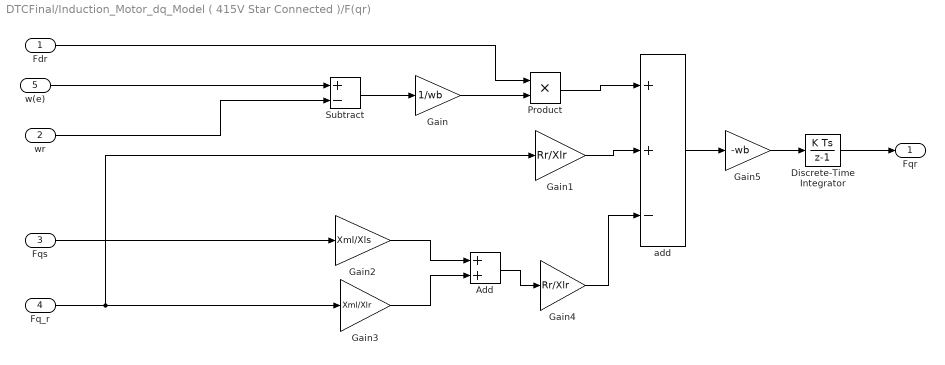
== system DTCFinal/Induction_Motor_dq_Model ( 415V Star Connected )/F(qr) ==
  Fdr : Inport
  wr : Inport  Port=2
  Fqs : Inport  Port=3
  Fq_r : Inport  Port=4
  w(e) : Inport  Port=5
  Add : Sum
  Discrete-Time Integrator : DiscreteIntegrator  InitialConditionSetting=State (most efficient)  SampleTime=Ts  ICPrevOutput=DiscIntNeverNeededParam  ICPrevScaledInput=DiscIntNeverNeededParam
  Gain : Gain  Gain=1/wb
  Gain1 : Gain  Gain=Rr/Xlr
  Gain2 : Gain  Gain=Xml/Xls
  Gain3 : Gain  Gain=Xml/Xlr
  Gain4 : Gain  Gain=Rr/Xlr
  Gain5 : Gain  Gain=-wb
  Product : Product
  Subtract : Sum  Inputs=+-
  add : Sum  Inputs=++-
  Fqr : Outport
  wires:
  Product/1 -> add/1
  Fdr/1 -> Product/1
  Fq_r/1 -> Gain1/1, Gain3/1
  Gain4/1 -> add/3
  Gain1/1 -> add/2
  wr/1 -> Subtract/2
  Gain/1 -> Product/2
  Gain3/1 -> Add/2
  Gain2/1 -> Add/1
  Fqs/1 -> Gain2/1
  Add/1 -> Gain4/1
  Subtract/1 -> Gain/1
  w(e)/1 -> Subtract/1
  add/1 -> Gain5/1
  Gain5/1 -> Discrete-Time Integrator/1
  Discrete-Time Integrator/1 -> Fqr/1

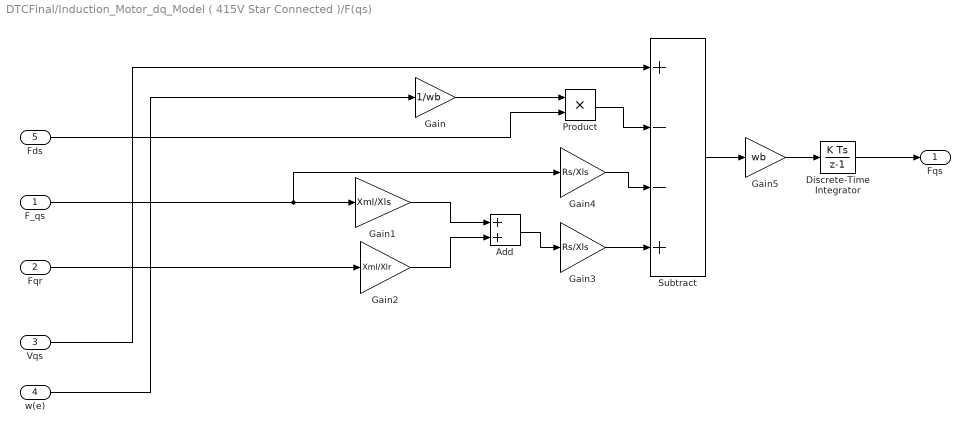
== system DTCFinal/Induction_Motor_dq_Model ( 415V Star Connected )/F(qs) ==
  F_qs : Inport
  Fqr : Inport  Port=2
  Vqs : Inport  Port=3
  "w(e) " : Inport  Port=4
  Fds : Inport  Port=5
  Add : Sum
  Discrete-Time Integrator : DiscreteIntegrator  InitialConditionSetting=State (most efficient)  SampleTime=Ts  ICPrevOutput=DiscIntNeverNeededParam  ICPrevScaledInput=DiscIntNeverNeededParam
  Gain : Gain  Gain=1/wb
  Gain1 : Gain  Gain=Xml/Xls
  Gain2 : Gain  Gain=Xml/Xlr
  Gain3 : Gain  Gain=Rs/Xls
  Gain4 : Gain  Gain=Rs/Xls
  Gain5 : Gain  Gain=wb
  Product : Product
  Subtract : Sum  Inputs=+--+
  Fqs : Outport
  wires:
  "w(e) "/1 -> Gain/1
  Fqr/1 -> Gain2/1
  Gain1/1 -> Add/1
  F_qs/1 -> Gain4/1, Gain1/1
  Gain4/1 -> Subtract/3
  Gain3/1 -> Subtract/4
  Add/1 -> Gain3/1
  Fds/1 -> Product/2
  Product/1 -> Subtract/2
  Gain5/1 -> Discrete-Time Integrator/1
  Subtract/1 -> Gain5/1
  Discrete-Time Integrator/1 -> Fqs/1
  Gain2/1 -> Add/2
  Vqs/1 -> Subtract/1
  Gain/1 -> Product/1

== system DTCFinal/Induction_Motor_dq_Model ( 415V Star Connected )/I(dr) ==
  "Fdr " : Inport
  Fmd : Inport  Port=2
  Gain : Gain  Gain=1/Xlr
  Subtract : Sum  Inputs=+-
  Iqs : Outport
  wires:
  Gain/1 -> Iqs/1
  Subtract/1 -> Gain/1
  "Fdr "/1 -> Subtract/1
  Fmd/1 -> Subtract/2

== system DTCFinal/Induction_Motor_dq_Model ( 415V Star Connected )/I(ds) ==
  "Fds " : Inport
  Fmd : Inport  Port=2
  Gain : Gain  Gain=1/Xls
  Subtract : Sum  Inputs=+-
  Ids : Outport
  wires:
  Gain/1 -> Ids/1
  Subtract/1 -> Gain/1
  "Fds "/1 -> Subtract/1
  Fmd/1 -> Subtract/2

== system DTCFinal/Induction_Motor_dq_Model ( 415V Star Connected )/I(qr) ==
  "Fqr " : Inport
  Fmq : Inport  Port=2
  Gain : Gain  Gain=1/Xlr
  Subtract : Sum  Inputs=+-
  Iqr : Outport
  wires:
  Fmq/1 -> Subtract/2
  "Fqr "/1 -> Subtract/1
  Subtract/1 -> Gain/1
  Gain/1 -> Iqr/1

== system DTCFinal/Induction_Motor_dq_Model ( 415V Star Connected )/I(qs) ==
  "Fqs " : Inport
  Fmq : Inport  Port=2
  Gain : Gain  Gain=1/Xls
  Subtract : Sum  Inputs=+-
  Iqs : Outport
  wires:
  Fmq/1 -> Subtract/2
  "Fqs "/1 -> Subtract/1
  Subtract/1 -> Gain/1
  Gain/1 -> Iqs/1

== system DTCFinal/Induction_Motor_dq_Model ( 415V Star Connected )/Wr(elec.) ==
  T(e) : Inport
  T(L) : Inport  Port=2
  In1 : Inport  Port=3
  Add : Sum  Inputs=+--
  Constant1 : Constant  Value=0.005
  Discrete-Time Integrator : DiscreteIntegrator  InitialConditionSetting=State (most efficient)  SampleTime=Ts  ICPrevOutput=DiscIntNeverNeededParam  ICPrevScaledInput=DiscIntNeverNeededParam
  Gain : Gain  Gain=P/(2*J)
  Product : Product
  wr : Outport
  wires:
  Discrete-Time Integrator/1 -> wr/1
  Gain/1 -> Discrete-Time Integrator/1
  Add/1 -> Gain/1
  T(L)/1 -> Add/2
  T(e)/1 -> Add/1
  In1/1 -> Product/1
  Product/1 -> Add/3
  Constant1/1 -> Product/2

== system DTCFinal/Induction_Motor_dq_Model ( 415V Star Connected )/conversion to syn frame  ==
  Vas : Inport
  Vbs : Inport  Port=2
  Vcs : Inport  Port=3
  "Theta( e ) (in rad.) " : Inport  Port=4
  2 Ph - 2Ph ( syn. rotating frame ) : Subsystem
  3Ph-2Ph conversion (Stationary Frame) : Subsystem
  Scope : Scope  NumInputPorts=2
  Scope1 : Scope
  Vds : Outport
  Vqs : Outport  Port=2
  wires:
  Vas/1 -> 3Ph-2Ph conversion (Stationary Frame)/1(Vas)
  Vcs/1 -> 3Ph-2Ph conversion (Stationary Frame)/3(Vcs)
  Vbs/1 -> 3Ph-2Ph conversion (Stationary Frame)/2(Vbs)
  2 Ph - 2Ph ( syn. rotating frame )/1(Vds) -> Scope/1, Vds/1
  "Theta( e ) (in rad.) "/1 -> Scope1/1, 2 Ph - 2Ph ( syn. rotating frame )/3("Theta( e) (in rad.) ")
  2 Ph - 2Ph ( syn. rotating frame )/2("Vqs ") -> Scope/2, Vqs/1
  3Ph-2Ph conversion (Stationary Frame)/2(Vdss) -> 2 Ph - 2Ph ( syn. rotating frame )/1(Vdss)
  3Ph-2Ph conversion (Stationary Frame)/1(Vqss) -> 2 Ph - 2Ph ( syn. rotating frame )/2(Vqss)

== system DTCFinal/Two- level Inverter /Subsystem ==
  Pulse A : Inport
  Pulse B : Inport  Port=2
  Pulse C : Inport  Port=3
  Phase Leg a : Switch  Criteria=u2 > Threshold  Threshold=0.5
  Phase leg b : Switch  Criteria=u2 > Threshold  Threshold=0.5
  "Phase leg c " : Switch  Criteria=u2 > Threshold  Threshold=0.5
  c : Constant  Value=0.5*Vdc
  c1 : Constant  Value=-0.5*Vdc
  c2 : Constant  Value=0.5*Vdc
  c3 : Constant  Value=-0.5*Vdc
  c4 : Constant  Value=0.5*Vdc
  c5 : Constant  Value=-0.5*Vdc
  Out1 : Outport
  Out2 : Outport  Port=2
  Out3 : Outport  Port=3
  wires:
  c2/1 -> Phase leg b/1
  c1/1 -> Phase Leg a/3
  Pulse C/1 -> "Phase leg c "/2
  Pulse A/1 -> Phase Leg a/2
  Pulse B/1 -> Phase leg b/2
  c4/1 -> "Phase leg c "/1
  Phase leg b/1 -> Out2/1
  Phase Leg a/1 -> Out1/1
  c/1 -> Phase Leg a/1
  c3/1 -> Phase leg b/3
  c5/1 -> "Phase leg c "/3
  "Phase leg c "/1 -> Out3/1

== system DTCFinal/Induction_Motor_dq_Model ( 415V Star Connected )/conversion to syn frame /2 Ph - 2Ph ( syn. rotating frame ) ==
  Vdss : Inport
  Vqss : Inport  Port=2
  "Theta( e) (in rad.) " : Inport  Port=3
  Add : Sum
  Add1 : Sum  Inputs=+-
  Product{,1..3} (4 alike) : Product
  t : Trigonometry  Operator=cos
  t1 : Trigonometry
  t2 : Trigonometry  Operator=cos
  t3 : Trigonometry
  Vds : Outport
  "Vqs " : Outport  Port=2
  wires:
  t/1 -> Product/2
  Vdss/1 -> Product3/1, Product/1
  "Theta( e) (in rad.) "/1 -> t1/1, t/1, t3/1, t2/1
  Add/1 -> Vds/1
  Add1/1 -> "Vqs "/1
  Product/1 -> Add/1
  t1/1 -> Product1/2
  Product1/1 -> Add/2
  t2/1 -> Product2/2
  Product2/1 -> Add1/1
  t3/1 -> Product3/2
  Product3/1 -> Add1/2
  Vqss/1 -> Product2/1, Product1/1

== system DTCFinal/Induction_Motor_dq_Model ( 415V Star Connected )/conversion to syn frame /3Ph-2Ph conversion (Stationary Frame) ==
  Vas : Inport
  Vbs : Inport  Port=2
  Vcs : Inport  Port=3
  Add : Sum  Inputs=+++
  Add1 : Sum  Inputs=+++
  Gain : Gain
  Gain1 : Gain  Gain=-1/2
  Gain2 : Gain  Gain=-1/2
  Gain3 : Gain  Gain=0
  Gain4 : Gain  Gain=-1.7321/2
  Gain5 : Gain  Gain=1.7321/2
  Gain8 : Gain  Gain=2/3
  Gain9 : Gain  Gain=2/3
  Vqss : Outport
  Vdss : Outport  Port=2
  wires:
  Vbs/1 -> Gain4/1, Gain1/1
  Vas/1 -> Gain/1, Gain3/1
  Gain5/1 -> Add1/3
  Vcs/1 -> Gain5/1, Gain2/1
  Gain4/1 -> Add1/2
  Gain3/1 -> Add1/1
  Gain/1 -> Add/1
  Gain1/1 -> Add/2
  Add/1 -> Gain8/1
  Add1/1 -> Gain9/1
  Gain8/1 -> Vqss/1
  Gain9/1 -> Vdss/1
  Gain2/1 -> Add/3

== matlab function DTCFinal/DTC/Look-up Table (For V_selection) ==
  data: n input; d_psi input; v output; dm input
function v=V_selection(n,d_psi,dm)
v=0;

%SECTOR 1 :
if(n==1)&&(d_psi==1)&&(dm==1)
    v=2;
end;
if(n==1)&&(d_psi==1)&&(dm==0)
    v=7;
end;
if(n==1)&&(d_psi==1)&&(dm==-1)
    v=6;
end;
if(n==1)&&(d_psi==0)&&(dm==1)
    v=3;
end;
if(n==1)&&(d_psi==0)&&(dm==0)
    v=0;
end;
if(n==1)&&(d_psi==0)&&(dm==-1)
    v=5;
end;
%SECTOR 2 :
if(n==2)&&(d_psi==1)&&(dm==1)
    v=3;
end;
if(n==2)&&(d_psi==1)&&(dm==0)
    v=0;
end;
if(n==2)&&(d_psi==1)&&(dm==-1)
    v=1;
end;
if(n==2)&&(d_psi==0)&&(dm==1)
    v=4;
end;
if(n==2)&&(d_psi==0)&&(dm==0)
    v=7;
end;
if(n==2)&&(d_psi==0)&&(dm==-1)
    v=6;
end;
%SECTOR 3 :
if(n==3)&&(d_psi==1)&&(dm==1)
    v=4;
end;
if(n==3)&&(d_psi==1)&&(dm==0)
    v=7;
end;
if(n==3)&&(d_psi==1)&&(dm==-1)
    v=2;
end;
if(n==3)&&(d_psi==0)&&(dm==1)
    v=5;
end;
if(n==3)&&(d_psi==0)&&(dm==0)
    v=0;
end;
if(n==3)&&(d_psi==0)&&(dm==-1)
    v=1;
end;
%SECTOR 4 :
if(n==4)&&(d_psi==1)&&(dm==1)
    v=5;
end;
if(n==4)&&(d_psi==1)&&(dm==0)
    v=0;
end;
if(n==4)&&(d_psi==1)&&(dm==-1)
    v=3;
end;
if(n==4)&&(d_psi==0)&&(dm==1)
    v=6;
end;
if(n==4)&&(d_psi==0)&&(dm==0)
    v=7;
end;
if(n==4)&&(d_psi==0)&&(dm==-1)
    v=2;
end;
%SECTOR 5 :
if(n==5)&&(d_psi==1)&&(dm==1)
    v=6;
end;
if(n==5)&&(d_psi==1)&&(dm==0)
    v=7;
end;
if(n==5)&&(d_psi==1)&&(dm==-1)
    v=4;
end;
if(n==5)&&(d_psi==0)&&(dm==1)
    v=1;
end;
if(n==5)&&(d_psi==0)&&(dm==0)
    v=0;
end;
if(n==5)&&(d_psi==0)&&(dm==-1)
    v=3;
end;
%SECTOR 6 :
if(n==6)&&(d_psi==1)&&(dm==1)
    v=1;
end;
if(n==6)&&(d_psi==1)&&(dm==0)
    v=0;
end;
if(n==6)&&(d_psi==1)&&(dm==-1)
    v=5;
end;
if(n==6)&&(d_psi==0)&&(dm==1)
    v=2;
end;
if(n==6)&&(d_psi==0)&&(dm==0)
    v=7;
end;
if(n==6)&&(d_psi==0)&&(dm==-1)
    v=4;
end;

== matlab function DTCFinal/Flux Reference ==
  data: flux input; y output; Wr input
function y = fcn(flux,Wr)
Wbase = 314.1593;
if Wr>Wbase 
    y = flux*(Wbase/Wr);
else
    y = flux;
end

== matlab function DTCFinal/DTC/Speed,Torque,Flux,Sector Calculator/Voltage Transformation ==
  data: Ia input; Id output; Ib input; Ic input; Iq output
function [Id,Iq] = fcn(Ia,Ib,Ic)
Id=(2/3)*(Ia-(0.5*Ib)-(0.5*Ic));
Iq=(2/3)*(((nthroot(3,2))/2)*Ib-((nthroot(3,2))/2)*Ic);
end

== matlab function DTCFinal/DTC/Speed,Torque,Flux,Sector Calculator/Torque ==
  data: fluxd input; y output; iq input; fluxq input; id input
function y = fcn(fluxd,iq,fluxq,id)
P=4;
y= (3/4)*P*(fluxd*iq-fluxq*id);
end

== matlab function DTCFinal/DTC/Speed,Torque,Flux,Sector Calculator/Omega Dot ==
  data: Te input; y output; Tload input; Wr input
function y = fcn(Te,Tload,Wr)
Jm=0.1390; % Combined rotor and load inertia
C=0.005;
y= (1/Jm)*(Te-Tload-C*Wr);
end

== matlab function DTCFinal/DTC/Speed,Torque,Flux,Sector Calculator/Current Transformation ==
  data: Va input; Vd output; Vb input; Vc input; Vq output
function [Vd,Vq] = fcn(Va,Vb,Vc)
Vd=(2/3)*(Va-(0.5*Vb)-(0.5*Vc));
Vq=(2/3)*(((nthroot(3,2))/2)*Vb-((nthroot(3,2))/2)*Vc);
end

== matlab function DTCFinal/DTC/Speed,Torque,Flux,Sector Calculator/Sector Estimator ==
  data: Fluxd input; n output; Fluxq input; deta output
function [n,deta]=SECTOR(Fluxd,Fluxq)
n=0;
deta=0;
deta=atan2(Fluxq,Fluxd);
if(deta>=-pi/6)&&(deta<pi/6)
    n=1;
end;
if(deta>=pi/6)&&(deta<pi/2)
    n=2;
end;
if(deta>=pi/2)&&(deta<5*pi/6)
    n=3;
end;
if(deta>=5*pi/6)&&(deta<pi)
    n=4;
end;
if(deta>=-pi)&&(deta<-5*pi/6)
    n=4;
end;
if(deta>=-5*pi/6)&&(deta<-pi/2)
    n=5;
end;
if(deta>=-pi/2)&&(deta<-pi/6)
    n=6;
end;

== matlab function DTCFinal/DTC/Speed,Torque,Flux,Sector Calculator/Flux Calculation ==
  data: isd input; fsddot output; isq input; vsd input; vsq input; fsqdot output
function [fsddot,fsqdot] = fcn(isd,isq,vsd,vsq)
Rs = 4.1250; 




fsddot = (-Rs * isd) + vsd ; 

fsqdot = (-Rs * isq) + vsq ;
